simulink model "identif"  (R2022b)
settings: Solver=VariableStepAuto  StartTime=0.0  StopTime=5000  RelTol=1e-3
values from neighbouring files (symbols this model uses):
  A = X(:, i+1:j-1)' \ X(:, i:j-2)'    [identification.m]
  B = X(:, i+1:j-1)' \ U(:, i:j-2)'    [identification.m]
  C = Y(:, i:j-1)' \ X(:, i:j-1)'    [identification.m]
  dt = 20    [identification.m]
  n = 10    [identification.m]
settings Model: Creator=lyeromona522  LastModifiedBy=lyeromona522

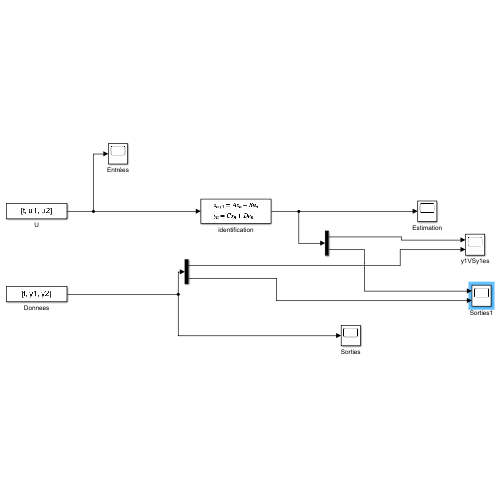
[thumbnail: Simulink's stored preview of the top-level diagram]
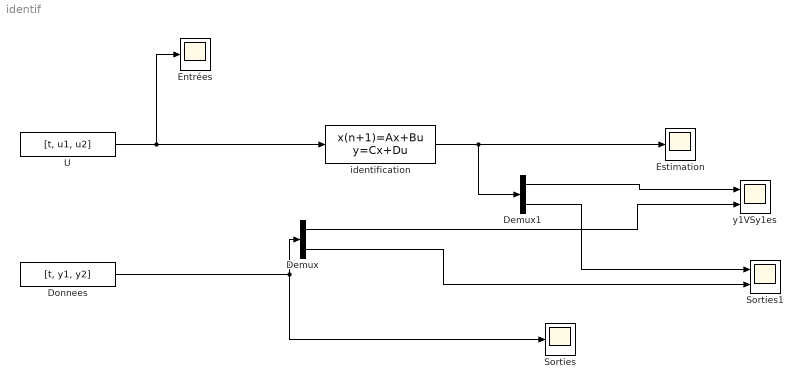
== system identif ==
  Demux : Demux  Outputs=2
  Demux1 : Demux  Outputs=2
  Donnees : FromWorkspace  VariableName=[t, y1, y2]  SampleTime=dt
  Entrées : Scope
  Estimation : Scope
  Sorties : Scope
  Sorties1 : Scope  NumInputPorts=2
  U : FromWorkspace  VariableName=[t, u1, u2]  SampleTime=dt
  identification : DiscreteStateSpace  A=A  B=B  C=C  D=zeros(2)  InitialCondition=rand(n,1)*0  SampleTime=dt
  y1VSy1es : Scope  NumInputPorts=2
  wires:
  U/1 -> identification/1, Entrées/1
  identification/1 -> Demux1/1, Estimation/1
  Donnees/1 -> Demux/1, Sorties/1
  Demux1/1 -> y1VSy1es/1
  Demux1/2 -> Sorties1/1
  Demux/1 -> y1VSy1es/2
  Demux/2 -> Sorties1/2
